simulink model "lmsblock"  (Simulink 2.20)
settings: Solver=ode1  StartTime=0.0  StopTime=1e10  RelTol=1e-3  AbsTol=1e-6
settings Model: ConsistencyChecking=off  RTWSystemTargetFile=rti1102.tlc  RTWPlaceOutputsASAP=off  RTWRetainRTWFile=on  RTWTemplateMakefile=rti1102.tmf  RTWMakeCommand=make_rti  RTWUserButton="RTI Settings...  rti_settings"  ExtModeMexFile=rti1102comm

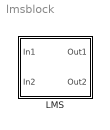
== system lmsblock ==
  LMS : Subsystem  mask(LMS){nnn=, mu=, Ts=}
      mask prompts: nnn "model structure"; mu "step length"; Ts "sampletime"
      mask Display:
      | text(0.1,0.25,'y')
      | text(0.1,0.85,'u')
      | text(0.8,0.8,'eps')
      | text(0.7,0.2,'threc')

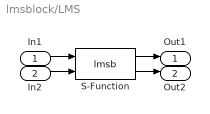
== system lmsblock/LMS ==
  In1 : Inport  Port=1  PortWidth=-1  SampleTime=-1
  In2 : Inport  Port=2  PortWidth=-1  SampleTime=-1
  S-Function : S-Function  FunctionName=lmsb  Parameters=nnn mu Ts  PortCounts=[]  SFunctionModules=''
  Out1 : Outport  Port=1  InitialOutput=0
  Out2 : Outport  Port=2  InitialOutput=0
  wires:
  S-Function/1 -> Out1/1
  In1/1 -> S-Function/1
  S-Function/2 -> Out2/1
  In2/1 -> S-Function/2
